simulink model "simulate_FM_Passband"  (R2021a)
settings: Solver=VariableStepAuto  StartTime=0.0  StopTime=0.1  RelTol=1e-3
InitFcn:
  | fs=4000;
  | frameSize=512;
libraries: simulink x1
settings Model: Creator=Byung-Jun Jang  LastModifiedBy=user
settings SolverCC: AlgebraicLoopSolver=TrustRegion
settings DataIOCC: ReturnWorkspaceOutputs=off
settings DebuggingCC: SFMachineParentedDataDiag=warning  ArithmeticOperatorsInVariantConditions=warning
settings SFSimCC: SimUseLocalCustomCode=off  CustomCodeUndefinedFunction=UseInterfaceOnly
settings RTWCC: RTWUseLocalCustomCode=off
settings CodeAppCC: StateflowObjectComments=on
settings SimscapeCC: SimscapeNormalizeSystem=off

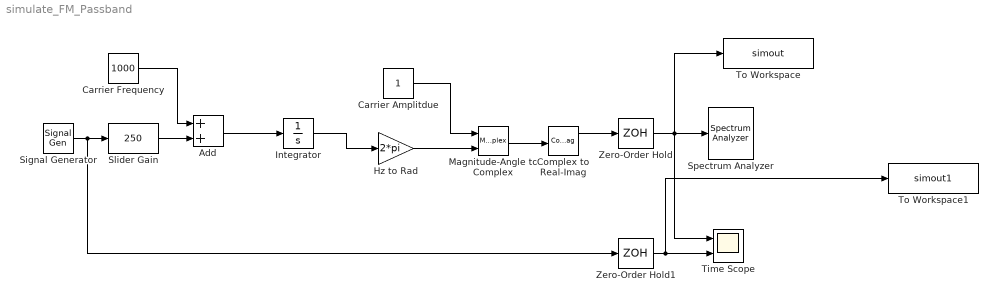
== system simulate_FM_Passband ==
  Add : Sum
  Carrier Amplitdue : Constant
  Carrier Frequency : Constant  Value=1000
  Complex to Real-Imag : ComplexToRealImag
  Hz to Rad : Gain  Gain=2*pi
  Integrator : Integrator
  Magnitude-Angle to Complex : MagnitudeAngleToComplex
  Signal Generator : SignalGenerator  Frequency=300
      settings: AttributesFormatString=|
      | Message
      | Signal
      | Generator
  Slider Gain : simulink/Math Operations/Slider Gain  gain=250  low=0  high=600
      settings: AttributesFormatString=|
      | Frequency
      | Sensitivity
  Spectrum Analyzer : SpectrumAnalyzer
  Time Scope : Scope  NumInputPorts=2
  To Workspace : ToWorkspace  VariableName=simout  SaveFormat=Timeseries  SampleTime=-1
  To Workspace1 : ToWorkspace  VariableName=simout1  SaveFormat=Timeseries  SampleTime=-1
  Zero-Order Hold : ZeroOrderHold  SampleTime=1/(fs*10)
  Zero-Order Hold1 : ZeroOrderHold  SampleTime=1/(fs*10)
  wires:
  Carrier Amplitdue/1 -> Magnitude-Angle to Complex/1
  Magnitude-Angle to Complex/1 -> Complex to Real-Imag/1
  Complex to Real-Imag/1 -> Zero-Order Hold/1
  Zero-Order Hold/1 -> To Workspace/1, Spectrum Analyzer/1, Time Scope/1
  Hz to Rad/1 -> Magnitude-Angle to Complex/2
  Signal Generator/1 -> Zero-Order Hold1/1, Slider Gain/1
  Slider Gain/1 -> Add/2
  Carrier Frequency/1 -> Add/1
  Add/1 -> Integrator/1
  Integrator/1 -> Hz to Rad/1
  Zero-Order Hold1/1 -> To Workspace1/1, Time Scope/2
